simulink model "PII_speed"  (Simulink 7.5)
settings: Solver=ode1  SolverMode=SingleTasking  StartTime=0.0  StopTime=Inf  FixedStep=ts  RelTol=1e-3
PostLoadFcn:
  | , if any(exist('dsrtsu_mdlpostloadfcn', 'file') == [2, 3, 6]), try dsrtsu_mdlpostloadfcn('Execute', bdroot); catch fprintf('Error in PostLoadFcn (dsrtsu_mdlpostloadfcn) for model "%s":\n %s\n', bdroot, lasterr); end, end,
values from neighbouring files (symbols this model uses):
  Amp = 0    [RUN.m]
  en = 0    [RUN.m]
  f = 0.20    (= 0.2)    [RUN.m]
  g = 1    [RUN.m]
  h1 = 31.3884    [RUN.m]
  h2 = -15.6627    [RUN.m]
  h3 = 199.8748    [RUN.m]
  h4 = -1.0744e+04    (= -10744)    [RUN.m]
  k1 = 4*ksi*omega*T1    (= 32.48)    [RUN.m]
  k2 = T1*Tc*((2*omega*omega)+(4*ksi*ksi*omega*omega)-(1/(T2*Tc))-(1/(T1*Tc)))    (= 3.06688)    [RUN.m]
  k3 = (T1*T2*Tc*4*ksi*(omega^3))-k1    (= -5.0512896)    [RUN.m]
  Ki = T1*T2*Tc*(omega^4)    (= 274.287104)    [RUN.m]
  kii = 660    [RUN.m]
  kpi = 2.0    (= 2)    [RUN.m]
  limit = 2    [RUN.m]
  nap = 0    [RUN.m]
  obc_del = 0.7    [RUN.m]
  obc_del2 = 1.3    [RUN.m]
  obc_en = 0    [RUN.m]
  obc_en1 = 0    [RUN.m]
  offset = 0    [RUN.m]
  res = 1    [RUN.m]
  res1 = 1    [RUN.m]
  start = 0    [RUN.m]
  T1 = 0.203    [RUN.m]
  T2 = 0.203    [RUN.m]
  Tc = 0.0026    [RUN.m]
  Tf = 0.01    [RUN.m]
  Ts_i = 0.0002    [RUN.m]
  Ts_w = 0.001    [RUN.m]
libraries: rtilib1103 x6, simulink_extras x1
settings Model: DSRTSU_INTERNAL_RTI_VER=400  DSRTSU_INTERNAL_RTI_TYPE=rti1103  Creator=lab108  LastModifiedBy=lab101  TunableVars=Amp,Q,Start,en,f,g,kii,kpi,n_max,n_min,nap,nb_nb,obc_del,obc_del2,obc_en,obc_en1,obc_poz,offset,p_gain,skal_u,start  TunableVarsStorageClass=Auto,Auto,Auto,Auto,Auto,Auto,Auto,Auto,Auto,Auto,Auto,Auto,Auto,Auto,Auto,Auto,Auto,Auto,Auto,Auto,Auto  TunableVarsTypeQualifier=,,,,,,,,,,,,,,,,,,,,  BufferReuse=off
settings OptimizationCC: BlockReduction=off  InlineParams=on  OptimizeBlockIOStorage=off  BufferReuse=off  ExpressionFolding=off  LocalBlockOutputs=off
settings DebuggingCC: StrictBusMsg=Warning
settings HardwareCC: ProdIntDivRoundTo=Zero  ProdEndianess=BigEndian  ProdHWDeviceType=Generic->Custom  TargetIntDivRoundTo=Zero  TargetEndianess=BigEndian  TargetHWDeviceType=Generic->Custom
settings RTWCC: SystemTargetFile=rti1103.tlc  MakeCommand=make_rti  TemplateMakefile=rti1103.tmf  Description=dSPACE DS1103 Hardware Platform  ProcessScript=rti1103_make_rtw_hook
settings STFCustomTargetCC: ParMdlRefBuildCompliant=on  GeneratePreprocessorConditionals=Disable all  SystemTargetFile=rti1103.tlc
settings GRTTargetCC: CompOptLevelCompliant=off  MatFileLogging=off  ExtModeMexFile=noextcomm
settings CustomProperty: DataType=RTWOptions_EnumType_D__dSPACE RCPHIL 73_matlab_rti1103_tlc_rti1103_1InitialSimState  Value=RUN
settings EnumStrPairs: String=RUN
settings SimEventsCC: propDiagAttribOutput=1  propDiagFcnCallOutput=1  propDiagStatOutput=0

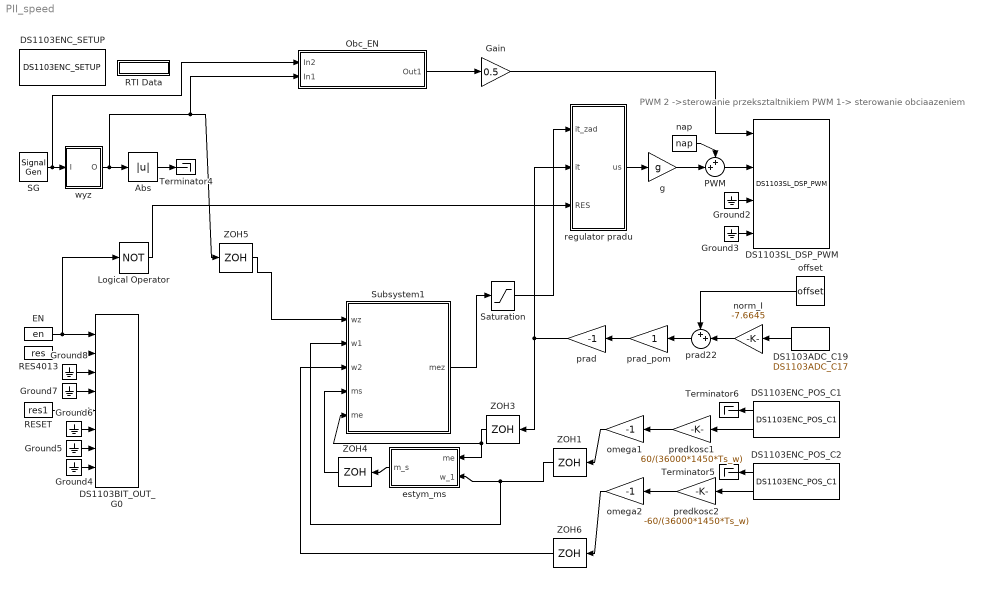
== system PII_speed ==
  note: PWM 2 ->sterowanie przeksztaltnikiem
      | PWM 1-> sterowanie obciaazeniem
  Abs : Abs  OutDataType=fixdt(1, 16)  OutScaling=2^0
  DS1103ADC_C19 : rtilib1103/DS1103 MASTER PPC/DS1103ADC_C17  SystemSampleTime=-1  ChannelNo=19  TimerAPreTrigger=0  Reserved2=[]  Reserved3=[]  Reserved4=[]  DialogFcn=gui1103adc  UnitName={ 'DS1103ADC_C' }  UnitValues={ 19 }  DSProperties=struct('RTI',struct('Version',uint32(1),'BlockType',struct('isSLSource',uint8(1),'isSLSink',uint8(0),'isHWSource',uint8(1),'isHWSink',uint8(0),'isSetup',uint8(0),'isInline',uint8(1),'isNonInline',uint8(0),'isInterrupt',uint8(0),'isChannelwise',uint8(1)),'IOBoardType','DS1103MASTER','UnitType','ADC','Identifier','ADC','DialogType','ML','BlockSet','NONE','SlaveProcessor','NONE'))
  DS1103BIT_OUT_G0 : rtilib1103/DS1103 MASTER PPC/DS1103BIT_OUT_G0  SystemSampleTime=-1  GroupNo=0  InitValue=[0 0 0 0 0 0 0 0]  TermMode=[1 1 1 1 1 1 1 1]  TermValue=[0 0 0 0 0 0 0 0]  Reserved1=[]  Reserved2=[]  Reserved3=[]  Reserved=[]  DialogFcn=gui1103bit_out  UnitName={ 'DS1103BIT_OUT_G'}  UnitValues={ 0 }  DSProperties=struct('RTI',struct('Version',uint32(1),'BlockType',struct('isSLSource',uint8(0),'isSLSink',uint8(1),'isHWSource',uint8(0),'isHWSink',uint8(1),'isSetup',uint8(0),'isInline',uint8(1),'isNonInline',uint8(0),'isInterrupt',uint8(0),'isChannelwise',uint8(0)),'IOBoardType','DS1103MASTER','UnitType','BIT','Identifier','BITOUT','DialogType','ML','BlockSet','NONE','SlaveProcessor','NONE'))
  DS1103ENC_POS_C1 : rtilib1103/DS1103 MASTER PPC/DS1103ENC_POS_C1  SystemSampleTime=-1  ChannelNo=1  PosValue=0  Reserved1=[]  Reserved2=[]  Reserved3=[]  Reserved4=[]  DialogFcn=gui1103enc_pos  UnitName={ 'DS1103ENC_POS_C' }  UnitValues={ 1 }  DSProperties=struct('RTI',struct('Version',uint32(1),'BlockType',struct('isSLSource',uint8(1),'isSLSink',uint8(0),'isHWSource',uint8(1),'isHWSink',uint8(0),'isSetup',uint8(0),'isInline',uint8(1),'isNonInline',uint8(0),'isInterrupt',uint8(0),'isChannelwise',uint8(1)),'IOBoardType','DS1103MASTER','UnitType','ENC','Identifier','ENCPOSCH','DialogType','ML','BlockSet','NONE','SlaveProcessor','NONE'))
  DS1103ENC_POS_C2 : rtilib1103/DS1103 MASTER PPC/DS1103ENC_POS_C1  SystemSampleTime=-1  ChannelNo=2  PosValue=0  Reserved1=[]  Reserved2=[]  Reserved3=[]  Reserved4=[]  DialogFcn=gui1103enc_pos  UnitName={ 'DS1103ENC_POS_C' }  UnitValues={2}  DSProperties=struct('RTI',struct('Version',uint32(1),'BlockType',struct('isSLSource',uint8(1),'isSLSink',uint8(0),'isHWSource',uint8(1),'isHWSink',uint8(0),'isSetup',uint8(0),'isInline',uint8(1),'isNonInline',uint8(0),'isInterrupt',uint8(0),'isChannelwise',uint8(1)),'IOBoardType','DS1103MASTER','UnitType','ENC','Identifier','ENCPOSCH','DialogType','ML','BlockSet','NONE','SlaveProcessor','NONE'))
  DS1103ENC_SETUP : rtilib1103/DS1103 MASTER PPC/DS1103ENC_SETUP  SystemSampleTime=-1  EncRange=2  Reserved1=[]  Reserved2=[]  Reserved3=[]  Reserved4=[]  DialogFcn=gui1103enc_setup  UnitName={ 'DS1103ENC_SETUP' }  UnitValues={ [] }  DSProperties=struct('RTI',struct('Version',uint32(1),'BlockType',struct('isSLSource',uint8(0),'isSLSink',uint8(0),'isHWSource',uint8(0),'isHWSink',uint8(0),'isSetup',uint8(0),'isInline',uint8(1),'isNonInline',uint8(0),'isInterrupt',uint8(0),'isChannelwise',uint8(0)),'IOBoardType','DS1103MASTER','UnitType','ENC','Identifier','ENCMASTER','DialogType','ML','BlockSet','NONE','SlaveProcessor','NONE'))
      settings: SignalType=[1 1 1 1 1 1 0]
  DS1103SL_DSP_PWM : rtilib1103/DS1103 SLAVE DSP/DS1103SL_DSP_PWM  SystemSampleTime=-1  Parameters=[]  TDef=[]  BoardType=[]  PwmMode=[]  Frequency=[]  InitValue=[]  TermMode=[]  TermValue=[]  Polarity=[]  DialogFcn=[]  Reserved1=[]  Reserved2=[]  Reserved3=[]  Reserved4=[]  Revision=[]  UnitName=[]  UnitValues=[]  DSProperties=struct('RTI',struct('Version',uint32(2),'BlockType',struct('isSLSource',uint8(0),'isSLSink',uint8(1),'isHWSource',uint8(0),'isHWSink',uint8(1),'isSetup',uint8(0),'isInline',uint8(1),'isNonInline',uint8(0),'isInterrupt',uint8(0),'isChannelwise',uint8(0)),'IOBoardType','DS1103SLAVE','UnitType','PWM','Identifier','PWM','DialogType','ML','BlockSet','NONE','SlaveProcessor','F240'))  RTIBlockInterface=struct('InputPortsActive',[1 1 1 1],'InputPortsWidth',int32([2 1 2 2]),'InputPortsName',{{['PWM Channel 1'],['PWM Channel 2'],['PWM Channel 3'],['PWM Channel 4']}},'IWork',{{{'',uint32(4)}}},'DialogFcn','rti1103slavepwmgui','InitLevel',1,'BlockDisplay',{{'','auto'}},'IconTransparency','on','MultiSFcn',4,'BlockName',struct('Token',{{'DS1103SL_DSP_PWM'}}))  RTIBlockParameters=struct('PWMSymmetryMode',{{1,'OFF',[]}},'PWMFrequency',{{'12000','OFF',[]}},'PWMPolarityMode',{{[1 1 1 1 1],'OFF',[]}},'ChannelNo',{{[1 2 3 4],'OFF',[]}},'SuspendModeInit',{{[1 0 1 1 1],'OFF',[]}},'TTLModeInit',{{[2 2 2 2 2],'OFF',[]}},'DutyCycleInitValueCh1',{{'0.5','OFF',[]}},'DutyCycleInitValueCh2',{{'0.5','OFF',[]}},'DutyCycleInitValueCh3',{{'0.5','OFF',[]}},'DutyCycleInitValueCh4',{{'0.5','OFF',[]}},'DutyCycleInitValueCh5',{{'0.5','OFF',[]}},'EnablePWMStop',{{[1 1 1 1 0],'OFF',[]}},'SuspendModeTerm',{{[1 0 1 1 1],'OFF',[]}},'TTLModeTerm',{{[2 2 2 2 2],'OFF',[]}},'DutyCycleTermValueCh1',{{'0.5','OFF',[]}},'DutyCycleTermValueCh2',{{'0.5','OFF',[]}},'DutyCycleTermValueCh3',{{'0.5','OFF',[]}},'DutyCycleTermValueCh4',{{'0.5','OFF',[]}},'DutyCycleTermValueCh5',{{'0.5','OFF',[]}},'TLCFileName',{{'rti1103pwm','OFF',[]}})  RTISFcnParameters=struct('PWMSymmetryMode','double','PWMFrequency','double','PWMPolarityMode','double','ChannelNo','double','SuspendModeInit','double','TTLModeInit','double','DutyCycleInitValueCh1','double','DutyCycleInitValueCh2','double','DutyCycleInitValueCh3','double','DutyCycleInitValueCh4','double','EnablePWMStop','double','SuspendModeTerm','double','TTLModeTerm','double','DutyCycleTermValueCh1','double','DutyCycleTermValueCh2','double','DutyCycleTermValueCh3','double','DutyCycleTermValueCh4','double','TLCFileName','char')  RTIBlockParaDefault=struct('PWMSymmetryMode',1,'PWMFrequency',100,'PWMPolarityMode',[1 1 1 1 1],'ChannelNo',[1 2 3 4],'SuspendModeInit',[1 1 1 1 1],'TTLModeInit',[2 2 2 2 2],'DutyCycleInitValueCh1',0.5,'DutyCycleInitValueCh2',0.5,'DutyCycleInitValueCh3',0.5,'DutyCycleInitValueCh4',0.5,'DutyCycleInitValueCh5',0.5,'EnablePWMStop',[1 1 1 1 0],'SuspendModeTerm',[1 1 1 1 1],'TTLModeTerm',[2 2 2 2 2],'DutyCycleTermValueCh1',0.5,'DutyCycleTermValueCh2',0.5,'DutyCycleTermValueCh3',0.5,'DutyCycleTermValueCh4',0.5,'DutyCycleTermValueCh5',0.5,'TLCFileName','rti1103pwm')
  EN : Constant  Value=en  OutDataTypeMode=boolean  OutDataType=fixdt(1, 16)  OutScaling=2^0  OutDataTypeStr=boolean
  Gain : Gain  Gain=0.5  ParameterDataType=sfix(16)  ParameterScaling=2^0  OutDataType=sfix(16)  OutScaling=2^0
  Ground{2..8} (7 alike) : Ground
  Logical Operator : Logic  Operator=NOT  AllPortsSameDT=off  OutDataTypeMode=boolean  LogicDataType=fixdt(0, 8)  OutDataTypeStr=boolean
  Obc_EN : Subsystem
  PWM : Sum  Inputs=++|  OutDataType=sfix(16)  OutScaling=2^0
  RES4013 : Constant  Value=res  OutDataTypeMode=boolean  OutDataType=fixdt(1, 16)  OutScaling=2^0  OutDataTypeStr=boolean
  RESET : Constant  Value=res1  OutDataTypeMode=boolean  OutDataType=fixdt(1, 16)  OutScaling=2^0  OutDataTypeStr=boolean
  RTI Data : Subsystem  Tag=struct('RTIDataServer',struct('RTIDataServerVs','2','RTIModelDescription','struct(''main'',''PII_speed'',''sub'','''',''isMp'',0)'))  LoadFcn="if exist('rtidc'), try,  rtidc('DataHostBlockClbLoad', gcbh); catch, disp(['Warning: ''LoadFcn'' for RTI Data block failed: ' lasterr]); end, end,"
      settings: CopyFcn="if exist('rtidc'), try,  rtidc('DataHostBlockClbCopy', gcbh); catch, disp(['Warning: ''CopyFcn'' for RTI Data block failed: ' lasterr]); end, end,"  DeleteFcn="if exist('rtidc'), try,  rtidc('DataHostBlockClbDelete', gcbh); catch, disp(['Warning: ''DeleteFcn'' for RTI Data block failed: ' lasterr]); end, end,"  ModelCloseFcn="if exist('rtidc'), try,  rtidc('DataHostBlockClbModelClose', gcbh); catch, disp(['Warning: ''ModelCloseFcn'' for RTI Data block failed: ' lasterr]); end, end,"  PreSaveFcn="if exist('rtidc'), try,  rtidc('DataHostBlockClbPreSave', gcbh); catch, disp(['Warning: ''PreSaveFcn'' for RTI Data block failed: ' lasterr]); end, end,"  PostSaveFcn="if exist('rtidc'), try,  rtidc('DataHostBlockClbPostSave', gcbh); catch, disp(['Warning: ''PostSaveFcn'' for RTI Data block failed: ' lasterr]); end, end,"  NameChangeFcn="if exist('rtidc'), try,  rtidc('DataHostBlockClbNameChange', gcbh); catch, disp(['Warning: ''NameChangeFcn'' for RTI Data block failed: ' lasterr]); end, end,"
      mask Type: RTI_DATA_HOST
      mask Description:
      | RTI Data Block.
      | This block is used by RTI to store internal model-dependent data.
      | Please keep this block on the root level of the model. Deleting this block will result in data loss.
      | 
      | NEVER DELETE OR COPY THIS BLOCK!
      mask Help:
      | RTI Data Block.
      | This block is used by RTI to store internal model-dependent data.
      | Please keep this block on the root level of the model. Deleting this block will result in data loss.
      | 
      | NEVER DELETE OR COPY THIS BLOCK!
      mask Display:
      | text(0.5, 0.5, 'RTI Data', 'HorizontalAlignment', 'center');
      | plot([1 0]);
  SG : SignalGenerator  WaveForm=square  Amplitude=Amp  Frequency=f
  Saturation : Saturate  UpperLimit=limit  LowerLimit=-limit
  Subsystem1 : Subsystem
  Terminator4 : Terminator
  Terminator5 : Terminator
  Terminator6 : Terminator
  ZOH{1,3..6} (5 alike) : ZeroOrderHold  SampleTime=Ts_w
  estym_ms : Subsystem
  g : Gain  Gain=g  ParameterDataType=fixdt(1, 16)  ParameterScaling=2^0  OutDataType=fixdt(1, 16)  OutScaling=2^0
  nap : Constant  Value=nap  OutDataType=sfix(16)  OutScaling=2^0
  norm_I : Gain  Gain=-7.6645  ParameterDataType=fixdt(1, 16)  ParameterScaling=2^0  OutDataType=fixdt(1, 16)  OutScaling=2^0
  offset : Constant  Value=offset  OutDataType=sfix(16)  OutScaling=2^0
  omega1 : Gain  Gain=-1  OutDataTypeMode=double  OutDataTypeStr=double  SampleTime=Ts_w  SaturateOnIntegerOverflow=on  ParamDataTypeStr=Inherit: Same as input
  omega2 : Gain  Gain=-1  OutDataTypeMode=double  OutDataTypeStr=double  SampleTime=Ts_w  SaturateOnIntegerOverflow=on  ParamDataTypeStr=Inherit: Same as input
  prad : Gain  Gain=-1  OutDataTypeMode=double  OutDataTypeStr=double  SampleTime=Ts_i  SaturateOnIntegerOverflow=on  ParamDataTypeStr=Inherit: Same as input
  prad22 : Sum  Inputs=++|  OutDataType=sfix(16)  OutScaling=2^0
  prad_pom : Gain  OutDataTypeMode=double  OutDataTypeStr=double  SampleTime=Ts_i  SaturateOnIntegerOverflow=on  ParamDataTypeStr=Inherit: Same as input
  predkosc1 : Gain  Gain=60/(36000*1450*Ts_w)  OutDataTypeMode=double  OutDataTypeStr=double  SampleTime=Ts_w  SaturateOnIntegerOverflow=on  ParamDataTypeStr=Inherit: Same as input
  predkosc2 : Gain  Gain=-60/(36000*1450*Ts_w)  OutDataTypeMode=double  OutDataTypeStr=double  SampleTime=Ts_w  SaturateOnIntegerOverflow=on  ParamDataTypeStr=Inherit: Same as input
  regulator pradu : Subsystem
  wyz : Subsystem
  wires:
  EN/1 -> DS1103BIT_OUT_G0/1, Logical Operator/1
  RESET/1 -> DS1103BIT_OUT_G0/5
  RES4013/1 -> DS1103BIT_OUT_G0/2
  DS1103ADC_C19/1 -> norm_I/1
  offset/1 -> prad22/1
  norm_I/1 -> prad22/2
  DS1103ENC_POS_C1/2 -> predkosc1/1
  prad22/1 -> prad_pom/1
  DS1103ENC_POS_C2/2 -> predkosc2/1
  nap/1 -> PWM/1
  regulator pradu/1(us) -> g/1
  PWM/1 -> DS1103SL_DSP_PWM/2
  g/1 -> PWM/2
  SG/1 -> wyz/1(I), Obc_EN/1(In2)
  predkosc2/1 -> omega2/1
  predkosc1/1 -> omega1/1
  wyz/1(O) -> Abs/1, Obc_EN/2(In1), ZOH5/1
  Ground2/1 -> DS1103SL_DSP_PWM/3
  Ground3/1 -> DS1103SL_DSP_PWM/4
  Ground4/1 -> DS1103BIT_OUT_G0/8
  Ground5/1 -> DS1103BIT_OUT_G0/7
  Ground6/1 -> DS1103BIT_OUT_G0/6
  Ground7/1 -> DS1103BIT_OUT_G0/4
  Ground8/1 -> DS1103BIT_OUT_G0/3
  Abs/1 -> Terminator4/1
  DS1103ENC_POS_C2/1 -> Terminator5/1
  DS1103ENC_POS_C1/1 -> Terminator6/1
  Logical Operator/1 -> regulator pradu/3(RES)
  prad/1 -> regulator pradu/2(it), ZOH3/1
  Obc_EN/1(Out1) -> Gain/1
  Gain/1 -> DS1103SL_DSP_PWM/1
  ZOH3/1 -> estym_ms/1(me), Subsystem1/5(me)
  omega1/1 -> ZOH1/1
  ZOH1/1 -> estym_ms/2(w_1), Subsystem1/2(w1)
  prad_pom/1 -> prad/1
  omega2/1 -> ZOH6/1
  estym_ms/1(m_s) -> ZOH4/1
  ZOH5/1 -> Subsystem1/1(wz)
  Saturation/1 -> regulator pradu/1(it_zad)
  Subsystem1/1(mez) -> Saturation/1
  ZOH6/1 -> Subsystem1/3(w2)
  ZOH4/1 -> Subsystem1/4(ms)

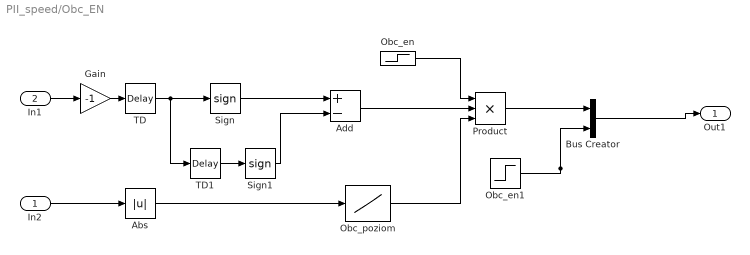
== system PII_speed/Obc_EN ==
  In2 : Inport
  In1 : Inport  Port=2
  Abs : Abs  OutDataType=fixdt(1, 16)  OutScaling=2^0
  Add : Sum  Inputs=+-  OutDataType=fixdt(1, 16)  OutScaling=2^-10
  Bus Creator : BusCreator  Inputs=2
  Gain : Gain  Gain=-1  ParameterDataType=sfix(16)  ParameterScaling=2^0  OutDataType=sfix(16)  OutScaling=2^0
  Obc_en : Step  Time=0  After=obc_en  SampleTime=0
  Obc_en1 : Step  Time=0  After=obc_en1  SampleTime=0
  Obc_poziom : Lookup  InputValues=[0,0.25,0.3,0.4,0.5,0.6,0.75,1]  Table=[-1,-1,-0.78,-0.4,-0.3,-0.24,-0.18,-0.13]  OutDataType=fixdt(1, 16)  OutScaling=2^0
  Product : Product  Inputs=3  OutDataType=sfix(16)  OutScaling=2^0  RndMeth=Zero
  Sign : Signum
  Sign1 : Signum
  TD : TransportDelay  DelayTime=obc_del  BufferSize=60000
  TD1 : TransportDelay  DelayTime=obc_del2  BufferSize=60000
  Out1 : Outport
  wires:
  Obc_en/1 -> Product/1
  Product/1 -> Bus Creator/1
  In1/1 -> Gain/1
  Bus Creator/1 -> Out1/1
  TD/1 -> Sign/1, TD1/1
  Sign/1 -> Add/1
  Gain/1 -> TD/1
  TD1/1 -> Sign1/1
  Sign1/1 -> Add/2
  Add/1 -> Product/2
  Abs/1 -> Obc_poziom/1
  Obc_poziom/1 -> Product/3
  In2/1 -> Abs/1
  Obc_en1/1 -> Bus Creator/2

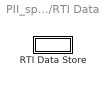
== system PII_speed/RTI Data ==
  RTI Data Store : Subsystem  Tag="struct('private',struct('version',struct('dsVer',uint32(2),'dsVerCreation',uint32(2),'RTI',struct('ver','6.4','type','RTI1103')),'access',struct('type','Model','isPerm',1,'created',['17-Sep-2010 12:08:45'],'modified',['17-Dec-2015 12:42:06'],'location','')),'public',struct('main',struct('data',[]),'sub',struct('name',{{'PII_speed'}},'data',{{struct('TH',struct('thTaskInfo',struct('taskType',{'TIMER','HWINT','TMRINT','SWINT','GLINT'},'tasksNumOf',{1,0,0,0,0},'srcIds',{{'TIMERA'},{},{},{},{}},'taskNames',{{['Timer Task 1']},{},{},{},{}})),'th_tc',struct('dataType','TASK','taskGroupId','','taskGroupList',{{}},'taskSchedulingPolicy','FCFS','taskType','TIMER','blkh',-1,'srcId','TIMERA','srcSgnName',['Timer A interrupt'],'srcCpuName','','taskName',['Timer Task 1  [0.0001] s'],'taskNameDisplayExt','','smplTime',0.0001,'smplTimeOffs',0,'hasFixedPriority',0,'priority',1,'hasFixedOvc',0,'ovcType',1,'ovcMax',1),'tc_th',struct('dataType','TASK','taskGroupId','','taskGroupList',{{}},'taskSchedulingPolicy','FCFS','taskType','TIMER','blkh',-1,'srcId','TIMERA','srcSgnName',['Timer A interrupt'],'srcCpuName','','taskName',['Timer Task 1  [0.0001] s'],'taskNameDisplayExt','','smplTime',0.0001,'smplTimeOffs',0,'hasFixedPriority',0,'priority',1,'hasFixedOvc',0,'ovcType',1,'ovcMax',1))}})))"
      mask Type: RTI_DATA_STORE
      mask Description:
      | RTI Data Store Block. This block is used by RTI to store internal model dependent data. Deleting this block will result in data loss.
      | 
      | NEVER DELETE, COPY, OR MODIFY THIS BLOCK!
      mask Help:
      | RTI Data Store Block. This block is used by RTI to store internal model dependent data. Deleting this block will result in data loss.
      | 
      | NEVER DELETE, COPY, OR MODIFY THIS BLOCK!
      mask Display: text(0.5, 0.5, ' ', 'HorizontalAlignment', 'center');

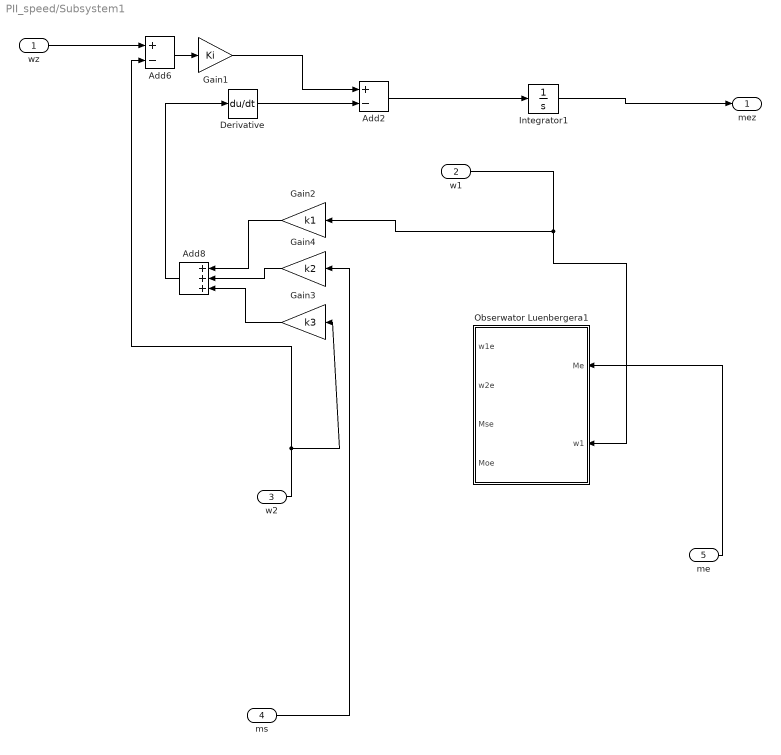
== system PII_speed/Subsystem1 ==
  wz : Inport
  w1 : Inport  Port=2
  w2 : Inport  Port=3
  ms : Inport  Port=4
  me : Inport  Port=5
  Add2 : Sum  Inputs=+-
  Add6 : Sum  Inputs=+-
  Add8 : Sum  Inputs=+++
  Derivative : Derivative
  Gain1 : Gain  Gain=Ki
  Gain2 : Gain  Gain=k1
  Gain3 : Gain  Gain=k3
  Gain4 : Gain  Gain=k2
  Integrator1 : Integrator  LimitOutput=on  UpperSaturationLimit=limit  LowerSaturationLimit=-limit
  Obserwator Luenbergera1 : Subsystem
  mez : Outport
  wires:
  Add8/1 -> Derivative/1
  Add6/1 -> Gain1/1
  Gain1/1 -> Add2/1
  w1/1 -> Gain2/1, Obserwator Luenbergera1/2(w1)
  Add2/1 -> Integrator1/1
  Gain2/1 -> Add8/1
  Gain4/1 -> Add8/2
  Gain3/1 -> Add8/3
  wz/1 -> Add6/1
  me/1 -> Obserwator Luenbergera1/1(Me)
  Integrator1/1 -> mez/1
  Derivative/1 -> Add2/2
  w2/1 -> Add6/2, Gain3/1
  ms/1 -> Gain4/1

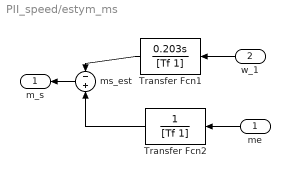
== system PII_speed/estym_ms ==
  me : Inport
  w_1 : Inport  Port=2
  Transfer Fcn1 : TransferFcn  Numerator=[0.203 0]  Denominator=[Tf 1]
  Transfer Fcn2 : TransferFcn  Denominator=[Tf 1]
  ms_est : Sum  Inputs=-+  OutDataType=sfix(16)  OutScaling=2^0
  m_s : Outport
  wires:
  ms_est/1 -> m_s/1
  me/1 -> Transfer Fcn2/1
  w_1/1 -> Transfer Fcn1/1
  Transfer Fcn2/1 -> ms_est/2
  Transfer Fcn1/1 -> ms_est/1

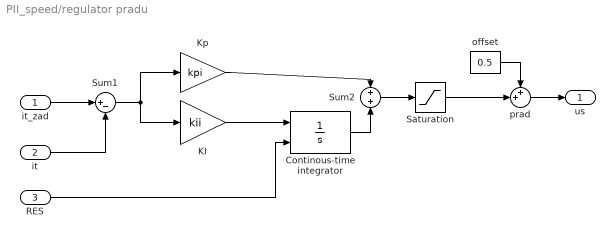
== system PII_speed/regulator pradu ==
  it_zad : Inport  SampleTime=Ts_i
  it : Inport  Port=2  SampleTime=Ts_i
  RES : Inport  Port=3  SampleTime=Ts_i
  Continous-time integrator : Integrator  ExternalReset=level  LimitOutput=on  UpperSaturationLimit=0.52  LowerSaturationLimit=-0.52
  KI : Gain  Gain=kii  SampleTime=Ts_i  SaturateOnIntegerOverflow=on  OutDataTypeStr=Inherit: Same as input  ParamDataTypeStr=Inherit: Same as input
  Kp : Gain  Gain=kpi  SampleTime=Ts_i  SaturateOnIntegerOverflow=on  OutDataTypeStr=Inherit: Same as input  ParamDataTypeStr=Inherit: Same as input
  Saturation : Saturate  UpperLimit=0.52  LowerLimit=-0.52  OutDataType=fixdt(1, 16)  OutScaling=2^0
  Sum1 : Sum  Inputs=|+-  SampleTime=Ts_i  SaturateOnIntegerOverflow=on  InputSameDT=on  OutDataTypeStr=Inherit: Same as first input
  Sum2 : Sum  SampleTime=Ts_i  SaturateOnIntegerOverflow=on  InputSameDT=on  OutDataTypeStr=Inherit: Same as first input
  offset : Constant  Value=0.5  OutDataType=sfix(16)  OutScaling=2^0  SampleTime=Ts_i
  prad : Sum  Inputs=++|  OutDataType=sfix(16)  OutScaling=2^0  SampleTime=Ts_i
  us : Outport
  wires:
  Kp/1 -> Sum2/1
  Sum2/1 -> Saturation/1
  Sum1/1 -> Kp/1, KI/1
  it/1 -> Sum1/2
  it_zad/1 -> Sum1/1
  RES/1 -> Continous-time integrator/2
  offset/1 -> prad/1
  prad/1 -> us/1
  KI/1 -> Continous-time integrator/1
  Continous-time integrator/1 -> Sum2/2
  Saturation/1 -> prad/2

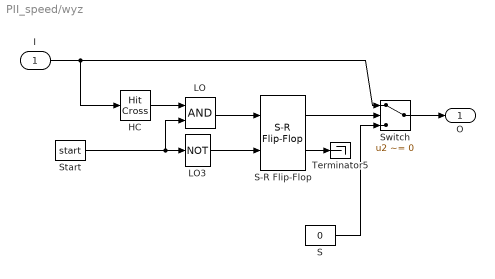
== system PII_speed/wyz ==
  I : Inport
  HC : HitCross  HitCrossingDirection=rising
  LO : Logic  AllPortsSameDT=off  OutDataTypeMode=boolean  LogicDataType=fixdt(0, 8)  OutDataTypeStr=boolean
  LO3 : Logic  Operator=NOT  AllPortsSameDT=off
  S : Constant  Value=0  OutDataTypeMode=boolean  OutDataTypeStr=boolean
  S-R Flip-Flop : simulink_extras/Flip Flops/S-R Flip-Flop  SystemSampleTime=-1  initial_condition=0
  Start : Constant  Value=start
  Switch : Switch  Criteria=u2 ~= 0  OutDataType=fixdt(1, 16)  OutScaling=2^0
  Terminator5 : Terminator
  O : Outport
  wires:
  Start/1 -> LO3/1, LO/2
  HC/1 -> LO/1
  LO/1 -> S-R Flip-Flop/1
  LO3/1 -> S-R Flip-Flop/2
  Switch/1 -> O/1
  S/1 -> Switch/3
  S-R Flip-Flop/1 -> Switch/2
  I/1 -> HC/1, Switch/1
  S-R Flip-Flop/2 -> Terminator5/1

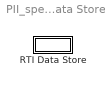
== system PII_speed/RTI Data/RTI Data Store ==
  RTI Data Store : Subsystem
      mask Type: RTI_DATA_STORE
      mask Description:
      | RTI Data Store Block. This block is used by RTI to store internal model dependent data. Deleting this block will result in data loss.
      | 
      | NEVER DELETE, COPY, OR MODIFY THIS BLOCK!
      mask Help:
      | RTI Data Store Block. This block is used by RTI to store internal model dependent data. Deleting this block will result in data loss.
      | 
      | NEVER DELETE, COPY, OR MODIFY THIS BLOCK!
      mask Display: text(0.5, 0.5, ' ', 'HorizontalAlignment', 'center');

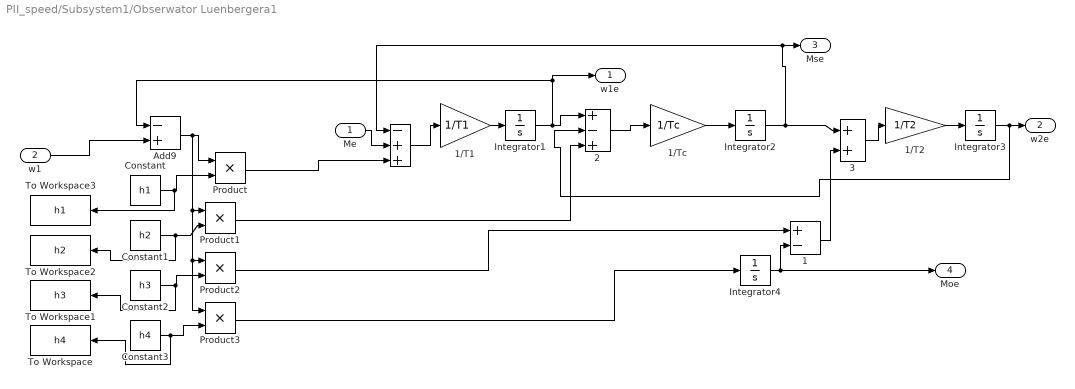
== system PII_speed/Subsystem1/Obserwator Luenbergera1 ==
  Me : Inport
  w1 : Inport  Port=2
  "  " : Sum  Inputs=-++
  "  1" : Sum  Inputs=+-
  "  2" : Sum  Inputs=+-+
  "  3" : Sum
  1/T1 : Gain  Gain=1/T1
  1/T2 : Gain  Gain=1/T2
  1/Tc : Gain  Gain=1/Tc
  Add9 : Sum  Inputs=-+
  Constant : Constant  Value=h1
  Constant1 : Constant  Value=h2
  Constant2 : Constant  Value=h3
  Constant3 : Constant  Value=h4
  Integrator{1..4} (4 alike) : Integrator
  Product{,1..3} (4 alike) : Product
  To Workspace : ToWorkspace  VariableName=h4  SampleTime=-1  SaveFormat=Array
      settings: MaxDataPoints=1
  To Workspace1 : ToWorkspace  VariableName=h3  SampleTime=-1  SaveFormat=Array
      settings: MaxDataPoints=1
  To Workspace2 : ToWorkspace  VariableName=h2  SampleTime=-1  SaveFormat=Array
      settings: MaxDataPoints=1
  To Workspace3 : ToWorkspace  VariableName=h1  SampleTime=-1  SaveFormat=Array
      settings: MaxDataPoints=1
  w1e : Outport
  w2e : Outport  Port=2
  Mse : Outport  Port=3
  Moe : Outport  Port=4
  wires:
  Product3/1 -> Integrator4/1
  Product2/1 -> "  1"/1
  Product1/1 -> "  2"/3
  Product/1 -> "  "/3
  Constant3/1 -> Product3/2, To Workspace/1
  Constant2/1 -> Product2/2, To Workspace1/1
  Constant1/1 -> Product1/2, To Workspace2/1
  Constant/1 -> Product/2, To Workspace3/1
  Add9/1 -> Product/1, Product1/1, Product2/1, Product3/1
  w1/1 -> Add9/2
  Integrator1/1 -> "  2"/1, w1e/1, Add9/1
  "  1"/1 -> "  3"/2
  Integrator4/1 -> "  1"/2, Moe/1
  Integrator3/1 -> w2e/1, "  2"/2
  "  2"/1 -> 1/Tc/1
  "  3"/1 -> 1/T2/1
  Integrator2/1 -> "  "/1, Mse/1, "  3"/1
  1/T2/1 -> Integrator3/1
  1/Tc/1 -> Integrator2/1
  1/T1/1 -> Integrator1/1
  "  "/1 -> 1/T1/1
  Me/1 -> "  "/2

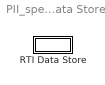
== system PII_speed/RTI Data/RTI Data Store/RTI Data Store ==
  RTI Data Store : Subsystem
      mask Type: RTI_DATA_STORE
      mask Description:
      | RTI Data Store Block. This block is used by RTI to store internal model dependent data. Deleting this block will result in data loss.
      | 
      | NEVER DELETE, COPY, OR MODIFY THIS BLOCK!
      mask Help:
      | RTI Data Store Block. This block is used by RTI to store internal model dependent data. Deleting this block will result in data loss.
      | 
      | NEVER DELETE, COPY, OR MODIFY THIS BLOCK!
      mask Display: text(0.5, 0.5, ' ', 'HorizontalAlignment', 'center');

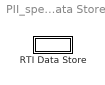
== system PII_speed/RTI Data/RTI Data Store/RTI Data Store/RTI Data Store ==
  RTI Data Store : Subsystem
      mask Type: RTI_DATA_STORE
      mask Description:
      | RTI Data Store Block. This block is used by RTI to store internal model dependent data. Deleting this block will result in data loss.
      | 
      | NEVER DELETE, COPY, OR MODIFY THIS BLOCK!
      mask Help:
      | RTI Data Store Block. This block is used by RTI to store internal model dependent data. Deleting this block will result in data loss.
      | 
      | NEVER DELETE, COPY, OR MODIFY THIS BLOCK!
      mask Display: text(0.5, 0.5, ' ', 'HorizontalAlignment', 'center');

== system PII_speed/RTI Data/RTI Data Store/RTI Data Store/RTI Data Store/RTI Data Store ==
